simulink model "SmartPCB_Reflow_AI_Model_FIXED"  (R2026a)
settings: Solver=ode45  StopTime=2400
libraries: slpidlib x1
settings Model: Creator=xianz  LastModifiedBy=xianz

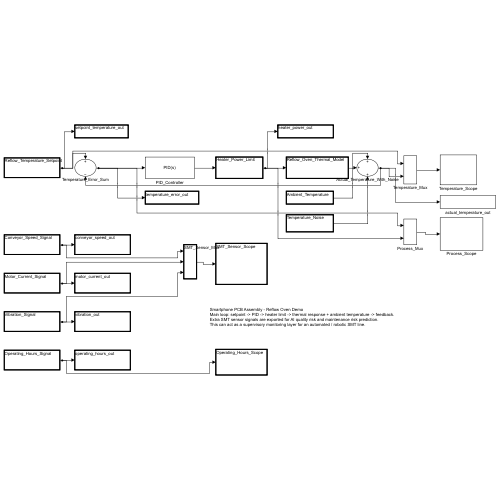
[thumbnail: Simulink's stored preview of the top-level diagram]
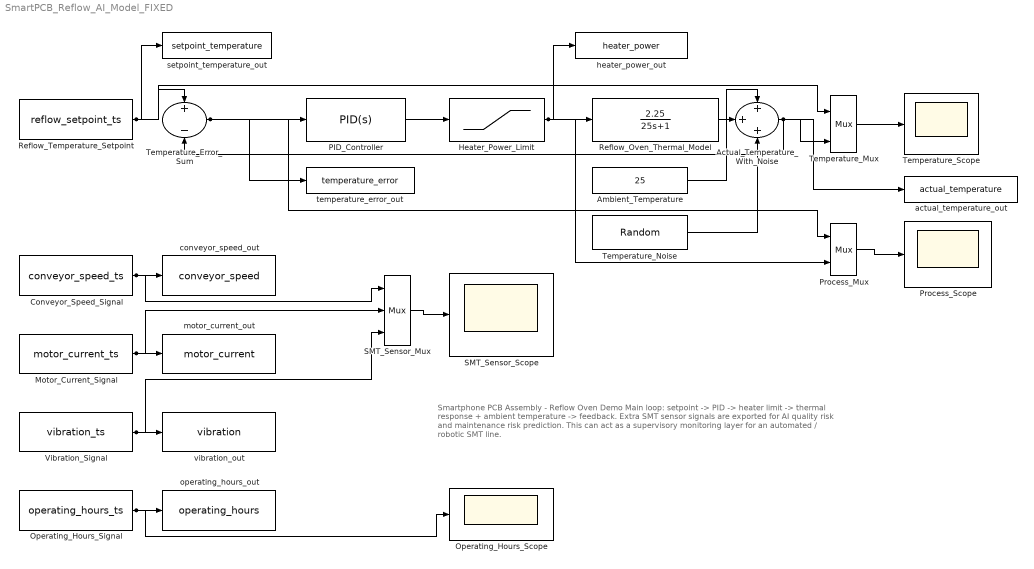
== system SmartPCB_Reflow_AI_Model_FIXED ==
  note: Smartphone PCB Assembly - Reflow Oven Demo
      | Main loop: setpoint -> PID -> heater limit -> thermal response + ambient temperature -> feedback.
      | Extra SMT sensor signals are exported for AI quality risk and maintenance risk prediction.
      | This can act as a supervisory monitoring layer for an automated / robotic SMT line.
  Actual_Temperature_With_Noise : Sum  Inputs=+++
  Ambient_Temperature : Constant  Value=25
  Conveyor_Speed_Signal : FromWorkspace  VariableName=conveyor_speed_ts
  Heater_Power_Limit : Saturate  UpperLimit=100  LowerLimit=0
  Motor_Current_Signal : FromWorkspace  VariableName=motor_current_ts
  Operating_Hours_Scope : Scope
  Operating_Hours_Signal : FromWorkspace  VariableName=operating_hours_ts
  PID_Controller : slpidlib/PID Controller  Controller=PID  Form=Parallel  TimeDomain=Continuous-time  UseExternalTs=off  SampleTime=-1  IntegratorMethod=Forward Euler  FilterMethod=Forward Euler  ControllerParametersSource=internal  P=1  I=1  UseKiTs=off  D=0  UseExternalDerivativeSource=off  N=100  UseFilter=on  TunerSelectOption=Transfer Function Based (PID Tuner App)  InitialConditionSource=internal  InitialConditionForIntegrator=0  InitialConditionForFilter=0  DifferentiatorICPrevScaledInput=0  ExternalReset=none  TrackingMode=off  Kt=1  LimitOutput=off  SatLimitsSource=internal  UpperSaturationLimit=inf  LowerSaturationLimit=-inf  LinearizeAsGain=on  AntiWindupMode=none  Kb=1  LimitIntegrator=off  UpperIntegratorSaturationLimit=inf  LowerIntegratorSaturationLimit=-inf  POutMin=[]  POutMax=[]  IOutMin=[]  IOutMax=[]  DOutMin=[]  DOutMax=[]  NOutMin=[]  NOutMax=[]  SumOutMin=[]  SumOutMax=[]  SaturationOutMin=[]  SaturationOutMax=[]  PParamMin=[]  PParamMax=[]  IParamMin=[]  IParamMax=[]  DParamMin=[]  DParamMax=[]  NParamMin=[]  NParamMax=[]  KbParamMin=[]  KbParamMax=[]  KtParamMin=[]  KtParamMax=[]  KbOutMin=[]  KbOutMax=[]  KtOutMin=[]  KtOutMax=[]  IntegratorOutMin=[]  IntegratorOutMax=[]  FilterOutMin=[]  FilterOutMax=[]  SumI1OutMin=[]  SumI1OutMax=[]  SumI2OutMin=[]  SumI2OutMax=[]  SumI3OutMin=[]  SumI3OutMax=[]  SumI4OutMin=[]  SumI4OutMax=[]  SumDOutMin=[]  SumDOutMax=[]  DifferentiatorOutMin=[]  DifferentiatorOutMax=[]  FilterDiffOutCoefMin=[]  FilterDiffOutCoefMax=[]  ReciprocalOutMin=[]  ReciprocalOutMax=[]  SumDenOutMin=[]  SumDenOutMax=[]  SumNumOutMin=[]  SumNumOutMax=[]  DivideOutMin=[]  DivideOutMax=[]  UdiffTsProdOutMin=[]  UdiffTsProdOutMax=[]  NTsProdOutMin=[]  NTsProdOutMax=[]  UintegralTsProdOutMin=[]  UintegralTsProdOutMax=[]  UngainTsProdOutMin=[]  UngainTsProdOutMax=[]  ClampingZeroOutDataTypeStr=Inherit: Inherit via back propagation  ClampingZeroOutMin=[]  ClampingZeroOutMax=[]  FilterDenConstantOutDataTypeStr=Inherit: Inherit via back propagation  FilterDenConstantOutMin=[]  FilterDenConstantOutMax=[]  PCopyOutDataTypeStr=Inherit: Inherit via back propagation  PCopyOutMin=[]  PCopyOutMax=[]  NCopyOutDataTypeStr=Inherit: Inherit via back propagation  NCopyOutMin=[]  NCopyOutMax=[]  IntegratorContinuousStateAttributes=''  IntegratorStateMustResolveToSignalObject=off  IntegratorRTWStateStorageClass=Auto  FilterContinuousStateAttributes=''  FilterStateMustResolveToSignalObject=off  FilterRTWStateStorageClass=Auto  ParallelPVariant=InternalParameters  IdealPVariant=Disabled  IVariant=InternalParameters  DVariant=InternalParameters  IntegratorVariant=Continuous  SatVariant=Disabled  AWVariant=Passthrough  PCopyVariant=Disabled  TRVariant=Disabled  FdbkBlocksVariant=Forward  IdealPFdbkVariant=Disabled  SatFdbkVariant=Disabled  DerivativeFilterVariant=ContFilter  NVariant=InternalParameters  NCopyVariant=Disabled  FilterICVariant=InternalICsFilter  IntegratorICVariant=InternalICs  ExternalResetVariant=Disabled  TRSumVariant=Passthrough  SumFdbkVariant=Disabled  SumVariant=Sum_PID  TsampFilterVariant=InternalTs  TsampNgainVariant=Passthrough  TsampIntegralVariant=Disabled_SignalSpec  ExternalSaturationOutDataTypeStr=Inherit: Same as second input  DerivativeSourceVariant=ErrorSignal  PreIntVariant=InternalPreInt
  Process_Mux : Mux  Inputs=2
  Process_Scope : Scope
  Reflow_Oven_Thermal_Model : TransferFcn  Numerator=[2.25]  Denominator=[25 1]
  Reflow_Temperature_Setpoint : FromWorkspace  VariableName=reflow_setpoint_ts
  SMT_Sensor_Mux : Mux  Inputs=3
  SMT_Sensor_Scope : Scope
  Temperature_Error_Sum : Sum  Inputs=+-
  Temperature_Mux : Mux  Inputs=2
  Temperature_Noise : RandomNumber  Variance=0.3  Seed=123  SampleTime=1
  Temperature_Scope : Scope
  Vibration_Signal : FromWorkspace  VariableName=vibration_ts
  actual_temperature_out : ToWorkspace  VariableName=actual_temperature  SaveFormat=Structure With Time  SampleTime=-1
  conveyor_speed_out : ToWorkspace  VariableName=conveyor_speed  SaveFormat=Structure With Time  SampleTime=-1
  heater_power_out : ToWorkspace  VariableName=heater_power  SaveFormat=Structure With Time  SampleTime=-1
  motor_current_out : ToWorkspace  VariableName=motor_current  SaveFormat=Structure With Time  SampleTime=-1
  operating_hours_out : ToWorkspace  VariableName=operating_hours  SaveFormat=Structure With Time  SampleTime=-1
  setpoint_temperature_out : ToWorkspace  VariableName=setpoint_temperature  SaveFormat=Structure With Time  SampleTime=-1
  temperature_error_out : ToWorkspace  VariableName=temperature_error  SaveFormat=Structure With Time  SampleTime=-1
  vibration_out : ToWorkspace  VariableName=vibration  SaveFormat=Structure With Time  SampleTime=-1
  wires:
  Reflow_Temperature_Setpoint/1 -> Temperature_Error_Sum/1, Temperature_Mux/1, setpoint_temperature_out/1
  Temperature_Error_Sum/1 -> PID_Controller/1, temperature_error_out/1, Process_Mux/1
  PID_Controller/1 -> Heater_Power_Limit/1
  Heater_Power_Limit/1 -> Reflow_Oven_Thermal_Model/1, heater_power_out/1, Process_Mux/2
  Reflow_Oven_Thermal_Model/1 -> Actual_Temperature_With_Noise/1
  Ambient_Temperature/1 -> Actual_Temperature_With_Noise/2
  Temperature_Noise/1 -> Actual_Temperature_With_Noise/3
  Actual_Temperature_With_Noise/1 -> Temperature_Error_Sum/2, Temperature_Mux/2, actual_temperature_out/1
  Temperature_Mux/1 -> Temperature_Scope/1
  Conveyor_Speed_Signal/1 -> conveyor_speed_out/1, SMT_Sensor_Mux/1
  Motor_Current_Signal/1 -> motor_current_out/1, SMT_Sensor_Mux/2
  Vibration_Signal/1 -> vibration_out/1, SMT_Sensor_Mux/3
  Operating_Hours_Signal/1 -> operating_hours_out/1, Operating_Hours_Scope/1
  Process_Mux/1 -> Process_Scope/1
  SMT_Sensor_Mux/1 -> SMT_Sensor_Scope/1
